simulink model "ClosedLoopNonlinearTuned"  (R2018a)
settings: Solver=VariableStepAuto  StartTime=0.0  StopTime=10.0  RelTol=1e-6
settings Model: Creator=melab2  LastModifiedBy=rahul

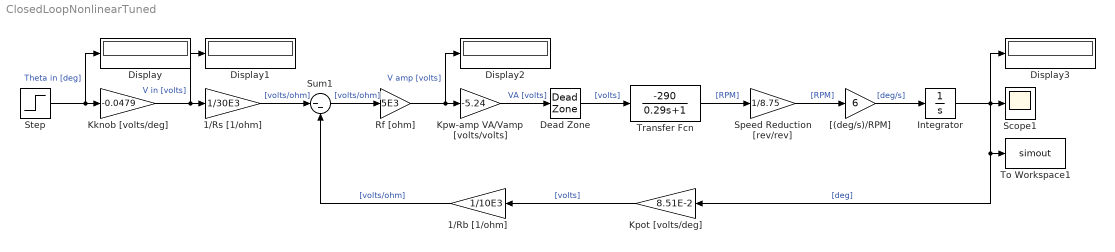
== system ClosedLoopNonlinearTuned ==
  1/Rb [1/ohm] : Gain  Gain=1/10E3
  1/Rs [1/ohm] : Gain  Gain=1/30E3
  "Dead Zone " : DeadZone  LowerValue=-1.9  UpperValue=1.9  SaturateOnIntegerOverflow=on
  Display{,1..3} (4 alike) : Display
  "Integrator " : Integrator
  Kknob [volts/deg] : Gain  Gain=-0.0479
  Kpot [volts/deg] : Gain  Gain=8.51E-2
  Kpw-amp VA/Vamp [volts/volts] : Gain  Gain=-5.24
  Rf [ohm] : Gain  Gain=5E3
  Scope1 : Scope
  Speed Reduction [rev/rev] : Gain  Gain=1/8.75
  Step : Step  After=200  SampleTime=0
  Sum1 : Sum  Inputs=|--
  To Workspace1 : ToWorkspace  VariableName=simout  SampleTime=-1
  "Transfer Fcn " : TransferFcn  Numerator=-290  Denominator=[0.29 1]
  "[(deg/s)/RPM]" : Gain  Gain=6
  wires:
  Rf [ohm]/1 -> Display2/1, Kpw-amp VA/Vamp [volts/volts]/1  "V amp [volts]"
  Sum1/1 -> Rf [ohm]/1  "[volts/ohm]"
  1/Rs [1/ohm]/1 -> Sum1/1  "[volts/ohm]"
  Kknob [volts/deg]/1 -> Display1/1, 1/Rs [1/ohm]/1  "V in [volts]"
  Step/1 -> Display/1, Kknob [volts/deg]/1  "Theta in [deg]"
  "Dead Zone "/1 -> "Transfer Fcn "/1  "[volts]"
  "Transfer Fcn "/1 -> Speed Reduction [rev/rev]/1  "[RPM]"
  Kpw-amp VA/Vamp [volts/volts]/1 -> "Dead Zone "/1  "VA [volts]"
  Speed Reduction [rev/rev]/1 -> "[(deg/s)/RPM]"/1  "[RPM]"
  "[(deg/s)/RPM]"/1 -> "Integrator "/1  "[deg/s]"
  1/Rb [1/ohm]/1 -> Sum1/2  "[volts/ohm]"
  Kpot [volts/deg]/1 -> 1/Rb [1/ohm]/1  "[volts]"
  "Integrator "/1 -> Display3/1, To Workspace1/1, Kpot [volts/deg]/1, Scope1/1  "[deg]"
